simulink model "modelo_practica0"  (R2022a)
settings: Solver=VariableStepAuto  StartTime=0.0  StopTime=10.0  RelTol=1e-3
undefined symbols (not defined in the file or in its folder): DiscIntNeverNeededParam
settings Model: Creator=Alba  LastModifiedBy=Alba

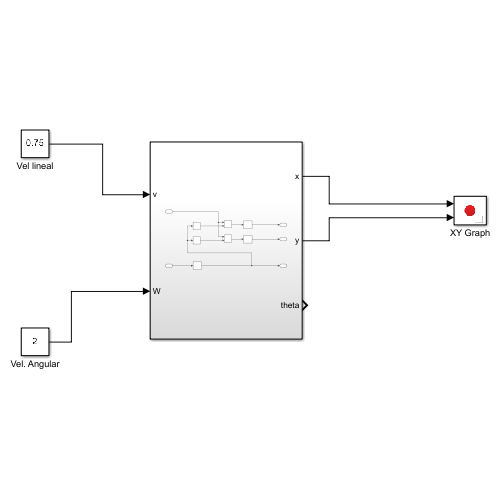
[thumbnail: Simulink's stored preview of the top-level diagram]
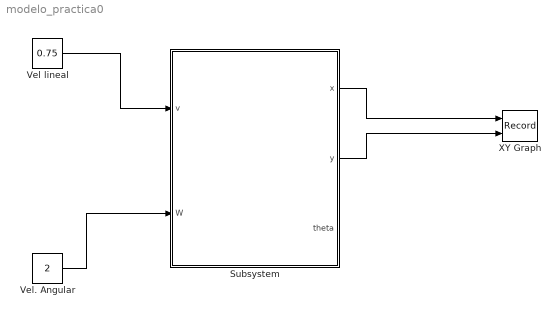
== system modelo_practica0 ==
  Subsystem : Subsystem
  Vel lineal : Constant  Value=0.75
  Vel. Angular : Constant  Value=2
  XY Graph : Record  FileSettingsInternal="{\"entries\":[{\"content\":{\"excelSettings\":{\"content\":{},\"type\":\"Streamout.ExcelSettings\"}},\"type\":\"Streamout.FileSettingStorage\",\"uuid\":\"a2675b60-8585-4ecd-8d4a-f731a51e02ec\"}],\"packageUris\":[\"http://schema.mathworks.com/mf0/streamout_blocks/R2020a\"],\"version\":\"1.0\"}"  Layout=[1 1]  SignalsInternal="{\"entries\":[{\"content\":{\"signals\":[{\"content\":{\"blockPath\":[\"modelo_practica0/XY Graph\"],\"channel\":[],\"dimensions\":[1],\"domain\":\"modelo_practica0/XY Graph\",\"lineColor\":\"#a2142f\",\"plots\":[1],\"port\":1,\"sid\":[],\"signalID\":17,\"signalName\":\"XY Graph:1\"},\"type\":\"RecordBlkView.Signal\",\"uuid\":\"70c4ea0e-4a97-4e72-a451-58d7ea2e1ab6\"},{\"content\":{\"blockPath\":[\"modelo_practica0/XY Graph\"],\"channel\":[],\"dimensions\":[1],\"domain\":\"modelo_practica0/XY Graph\",\"lineColor\":\"#139fff\",\"plots\":[1],\"port\":2,\"sid\":[],\"signalID\":20,\"signalName\":\"XY Graph:2\"},\"type\":\"RecordBlkView.Signal\",\"uuid\":\"153840da-0612-4c46-a2ad-d37790b90fa1\"}]},\"type\":\"RecordBlkView.InputSignals\",\"uuid\":\"621e361e-fa1c-4311-819a-4b7d32d077cd\"}],\"packageUris\":[\"http://schema.mathworks.com/mf0/streamout_blocks/R2020a\"],\"version\":\"1.0\"}"  VisualizationBindings="{\"xyplotplugin\":{\"info\":[{\"series\":[{\"bindingParametersList\":[{\"parameter\":\"X-Axis\",\"signalID\":17,\"signalName\":\"XY Graph:1\"},{\"parameter\":\"Y-Axis\",\"signalID\":20,\"signalName\":\"XY Graph:2\"}],\"seriesID\":7547}],\"subplotID\":1}]}}"  CompatibilityTag=XY
  wires:
  Vel lineal/1 -> Subsystem/1(v)
  Vel. Angular/1 -> Subsystem/2(W)
  Subsystem/1(x) -> XY Graph/1
  Subsystem/2(y) -> XY Graph/2

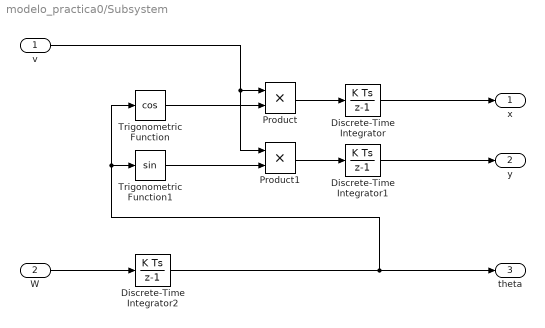
== system modelo_practica0/Subsystem ==
  v : Inport
  W : Inport  Port=2
  Discrete-Time Integrator : DiscreteIntegrator  SampleTime=-1  ICPrevOutput=DiscIntNeverNeededParam  ICPrevScaledInput=DiscIntNeverNeededParam
  Discrete-Time Integrator1 : DiscreteIntegrator  SampleTime=-1  ICPrevOutput=DiscIntNeverNeededParam  ICPrevScaledInput=DiscIntNeverNeededParam
  Discrete-Time Integrator2 : DiscreteIntegrator  SampleTime=-1  ICPrevOutput=DiscIntNeverNeededParam  ICPrevScaledInput=DiscIntNeverNeededParam
  Product : Product
  Product1 : Product
  Trigonometric Function : Trigonometry  Operator=cos
  Trigonometric Function1 : Trigonometry
  x : Outport
  y : Outport  Port=2
  theta : Outport  Port=3
  wires:
  Discrete-Time Integrator1/1 -> y/1
  v/1 -> Product1/1, Product/1
  W/1 -> Discrete-Time Integrator2/1
  Product/1 -> Discrete-Time Integrator/1
  Discrete-Time Integrator2/1 -> theta/1, Trigonometric Function/1, Trigonometric Function1/1
  Discrete-Time Integrator/1 -> x/1
  Trigonometric Function/1 -> Product/2
  Product1/1 -> Discrete-Time Integrator1/1
  Trigonometric Function1/1 -> Product1/2
